simulink model "Analise_Ganhos"  (R2021a)
settings: Solver=VariableStepAuto  StartTime=0.0  StopTime=1.015  MaxStep=1e-6  RelTol=1e-3
settings Model: Creator=migue  LastModifiedBy=migue

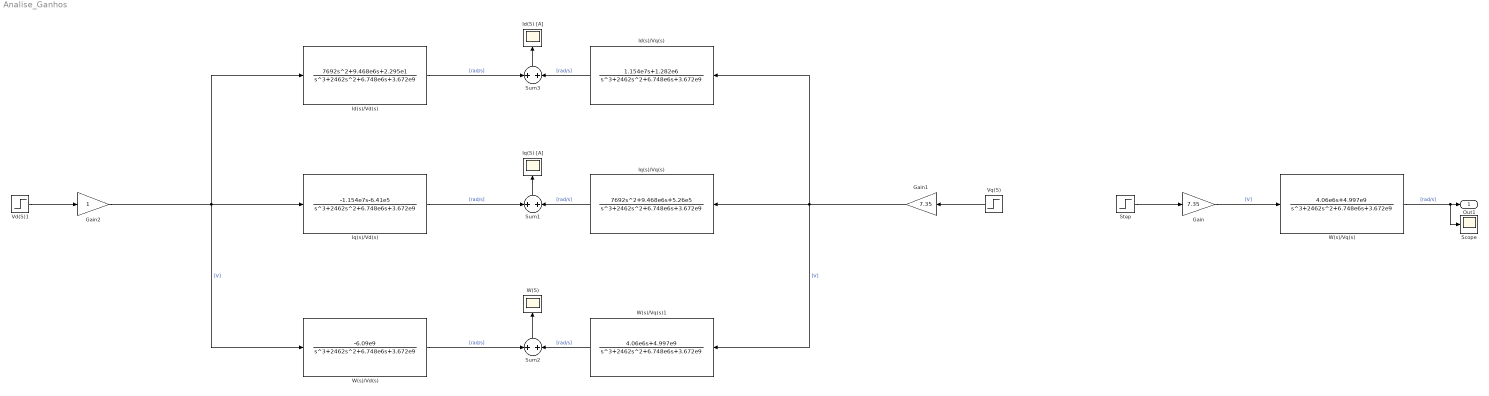
== system Analise_Ganhos ==
  Gain : Gain  Gain=7.35
  Gain1 : Gain  Gain=7.35
  Gain2 : Gain
  Id(S) [A] : Scope
  Id(s)/Vd(s) : TransferFcn  Numerator=[7692 9.468e6 2.295e1]  Denominator=[1 2462 6.748e6 3.672e9]
  Id(s)/Vq(s) : TransferFcn  Numerator=[1.154e7 1.282e6]  Denominator=[1 2462 6.748e6 3.672e9]
  Iq(S) [A] : Scope
  Iq(s)/Vd(s) : TransferFcn  Numerator=[-1.154e7 -6.41e5]  Denominator=[1 2462 6.748e6 3.672e9]
  Iq(s)/Vq(s) : TransferFcn  Numerator=[7692 9.468e6 5.26e5]  Denominator=[1 2462 6.748e6 3.672e9]
  Scope : Scope
  Step : Step  After=10  SampleTime=0
  Sum1 : Sum  Inputs=+|+
  Sum2 : Sum  Inputs=+|+
  Sum3 : Sum  Inputs=+|+
  Vd(S)1 : Step  After=0  SampleTime=0
  Vq(S) : Step  After=10  SampleTime=0
  W(S) : Scope
  W(s)/Vd(s) : TransferFcn  Numerator=[-6.09e9]  Denominator=[1 2462 6.748e6 3.672e9]
  W(s)/Vq(s) : TransferFcn  Numerator=[4.06e6 4.997e9]  Denominator=[1 2462 6.748e6 3.672e9]
  W(s)/Vq(s)1 : TransferFcn  Numerator=[4.06e6 4.997e9]  Denominator=[1 2462 6.748e6 3.672e9]
  Out1 : Outport
  wires:
  Step/1 -> Gain/1
  Gain/1 -> W(s)/Vq(s)/1  "[V]"
  W(s)/Vq(s)/1 -> Out1/1, Scope/1  "[rad/s]"
  Gain1/1 -> Id(s)/Vq(s)/1, Iq(s)/Vq(s)/1, W(s)/Vq(s)1/1  "[V]"
  Vq(S)/1 -> Gain1/1
  Sum2/1 -> W(S)/1
  W(s)/Vq(s)1/1 -> Sum2/2  "[rad/s]"
  Sum1/1 -> Iq(S) [A]/1
  Sum3/1 -> Id(S) [A]/1
  Iq(s)/Vq(s)/1 -> Sum1/2  "[rad/s]"
  Id(s)/Vq(s)/1 -> Sum3/2  "[rad/s]"
  Vd(S)1/1 -> Gain2/1
  Gain2/1 -> W(s)/Vd(s)/1, Iq(s)/Vd(s)/1, Id(s)/Vd(s)/1  "[V]"
  Iq(s)/Vd(s)/1 -> Sum1/1  "[rad/s]"
  Id(s)/Vd(s)/1 -> Sum3/1  "[rad/s]"
  W(s)/Vd(s)/1 -> Sum2/1  "[rad/s]"
